simulink model "QUESTION1_4"  (R2021a)
settings: Solver=VariableStepAuto  StartTime=0.0  StopTime=50  RelTol=1e-3
settings Model: Creator=user  LastModifiedBy=user

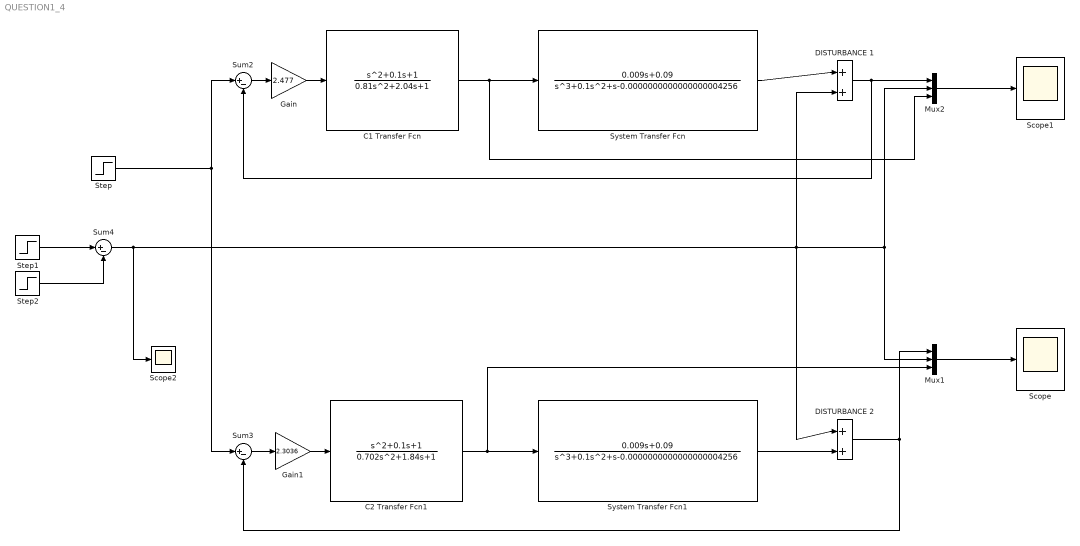
== system QUESTION1_4 ==
  C1 Transfer Fcn : TransferFcn  Numerator=[1 0.1 1]  Denominator=[0.81 2.04 1]
  C2 Transfer Fcn1 : TransferFcn  Numerator=[1 0.1 1]  Denominator=[0.702 1.84 1]
  DISTURBANCE 1 : Sum  Inputs=|++
  DISTURBANCE 2 : Sum  Inputs=|++
  Gain : Gain  Gain=2.477
  Gain1 : Gain  Gain=2.3036
  Mux1 : Mux  Inputs=3
  Mux2 : Mux  Inputs=3
  Scope : Scope
  Scope1 : Scope
  Scope2 : Scope
  Step : Step  SampleTime=0
  Step1 : Step  Time=22  SampleTime=0
  Step2 : Step  Time=24  SampleTime=0
  Sum2 : Sum  Inputs=|+-
  Sum3 : Sum  Inputs=|+-
  Sum4 : Sum  Inputs=|+-
  System Transfer Fcn : TransferFcn  Numerator=[0.009 0.09]  Denominator=[1 0.1 1 -0.0000000000000000004256]
  System Transfer Fcn1 : TransferFcn  Numerator=[0.009 0.09]  Denominator=[1 0.1 1 -0.0000000000000000004256]
  wires:
  Step/1 -> Sum3/1, Sum2/1
  C1 Transfer Fcn/1 -> System Transfer Fcn/1, Mux2/3
  C2 Transfer Fcn1/1 -> System Transfer Fcn1/1, Mux1/3
  Mux1/1 -> Scope/1
  Step1/1 -> Sum4/1
  Step2/1 -> Sum4/2
  Sum4/1 -> Scope2/1, Mux2/2, Mux1/2, DISTURBANCE 2/1, DISTURBANCE 1/2
  Mux2/1 -> Scope1/1
  System Transfer Fcn/1 -> DISTURBANCE 1/1
  DISTURBANCE 1/1 -> Mux2/1, Sum2/2
  DISTURBANCE 2/1 -> Sum3/2, Mux1/1
  System Transfer Fcn1/1 -> DISTURBANCE 2/2
  Gain/1 -> C1 Transfer Fcn/1
  Sum2/1 -> Gain/1
  Gain1/1 -> C2 Transfer Fcn1/1
  Sum3/1 -> Gain1/1
